simulink model "boggieDynamics2"  (R2022b)
settings: Solver=VariableStepAuto  StartTime=0.0  StopTime=10.0  RelTol=1e-3
values from neighbouring files (symbols this model uses):
  cg_nom = 0.567    [linealizacion_5gdl.m]    (also in linealizacion_HEMS.m)
undefined symbols (not defined in the file or in its folder): g, m, x_lev, x_lim, y_brk, y_lev, y_lim, z_brk, z_lev, z_lim
libraries: shared6dof x1
settings Model: Creator=USUARIO  LastModifiedBy=USUARIO

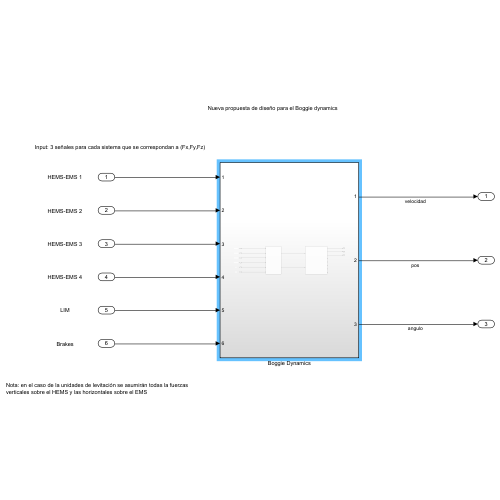
[thumbnail: Simulink's stored preview of the top-level diagram]
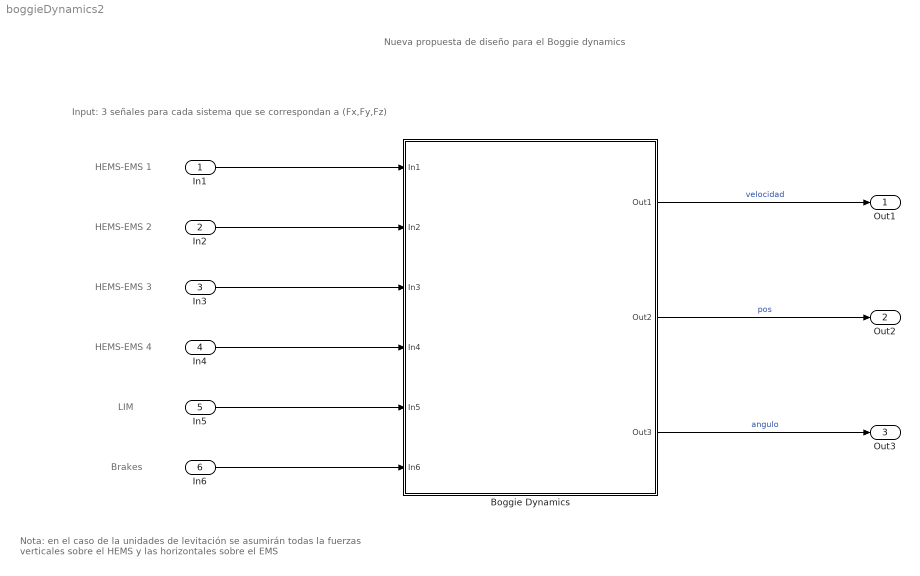
== system boggieDynamics2 ==
  note: Input: 3 señales para cada sistema que se correspondan a (Fx,Fy,Fz)
  note: Nueva propuesta de diseño para el Boggie dynamics
  note: HEMS-EMS 3
  note: Brakes
  note: HEMS-EMS 1
  note: LIM
  note: HEMS-EMS 4
  note: HEMS-EMS 2
  note: Nota: en el caso de la unidades de levitación se asumirán todas la fuerzas
      | verticales sobre el HEMS y las horizontales sobre el EMS
  In1 : Inport
  In2 : Inport  Port=2
  In3 : Inport  Port=3
  In4 : Inport  Port=4
  In5 : Inport  Port=5
  In6 : Inport  Port=6
  Boggie Dynamics : Subsystem
  Out1 : Outport
  Out2 : Outport  Port=2
  Out3 : Outport  Port=3
  wires:
  Boggie Dynamics/2(Out2) -> Out2/1  "pos"
  Boggie Dynamics/3(Out3) -> Out3/1  "angulo"
  Boggie Dynamics/1(Out1) -> Out1/1  "velocidad"
  In6/1 -> Boggie Dynamics/6(In6)
  In3/1 -> Boggie Dynamics/3(In3)
  In4/1 -> Boggie Dynamics/4(In4)
  In2/1 -> Boggie Dynamics/2(In2)
  In1/1 -> Boggie Dynamics/1(In1)
  In5/1 -> Boggie Dynamics/5(In5)

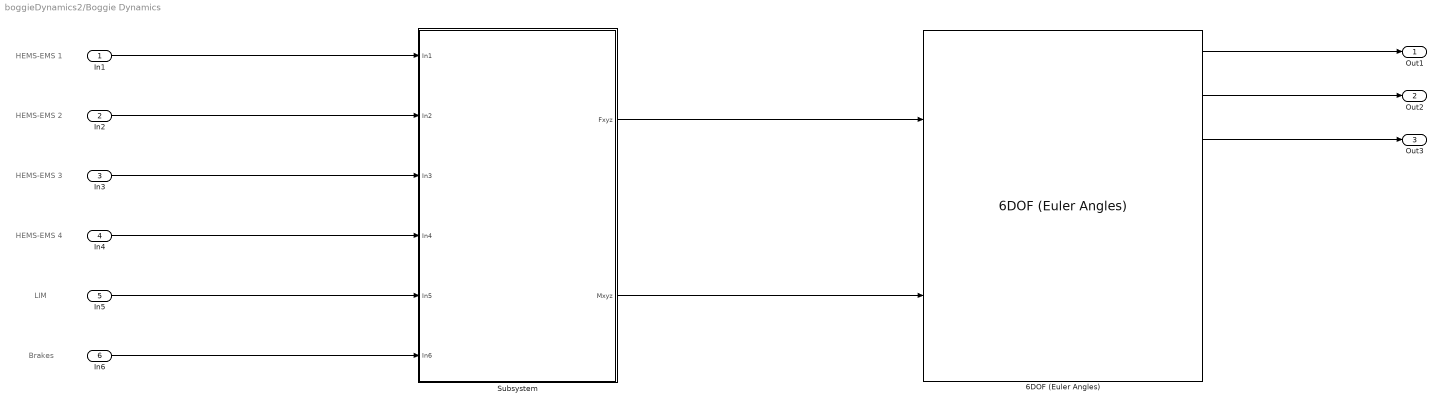
== system boggieDynamics2/Boggie Dynamics ==
  note: LIM
  note: HEMS-EMS 1
  note: HEMS-EMS 2
  note: HEMS-EMS 3
  note: HEMS-EMS 4
  note: Brakes
  In1 : Inport
  In2 : Inport  Port=2
  In3 : Inport  Port=3
  In4 : Inport  Port=4
  In5 : Inport  Port=5
  In6 : Inport  Port=6
  6DOF (Euler Angles) : shared6dof/6DOF (Euler Angles)  units=Metric (MKS)  mtype=Fixed  rep=Euler Angles  xme_0=[0 0 cg_nom]  Vm_0=[0 0 0]  eul_0=[0 0 0]  pm_0=[0 0 0]  mass_0=m  mass_e=0.5  mass_f=2.0  inertia=I  inertia_e=eye(3)  inertia_f=2*eye(3)  k_quat=1.0  vre_flag=on  abi_flag=off  aMode=0  xme_statename=''  Vm_statename=''  eul_statename=''  quat_statename=''  pm_statename=''  mass_statename=''
  Subsystem : Subsystem
  Out1 : Outport
  Out2 : Outport  Port=2
  Out3 : Outport  Port=3
  wires:
  6DOF (Euler Angles)/1 -> Out1/1
  6DOF (Euler Angles)/2 -> Out2/1
  6DOF (Euler Angles)/3 -> Out3/1
  In1/1 -> Subsystem/1(In1)
  In2/1 -> Subsystem/2(In2)
  In3/1 -> Subsystem/3(In3)
  In4/1 -> Subsystem/4(In4)
  In5/1 -> Subsystem/5(In5)
  In6/1 -> Subsystem/6(In6)
  Subsystem/1(Fxyz) -> 6DOF (Euler Angles)/1
  Subsystem/2(Mxyz) -> 6DOF (Euler Angles)/2

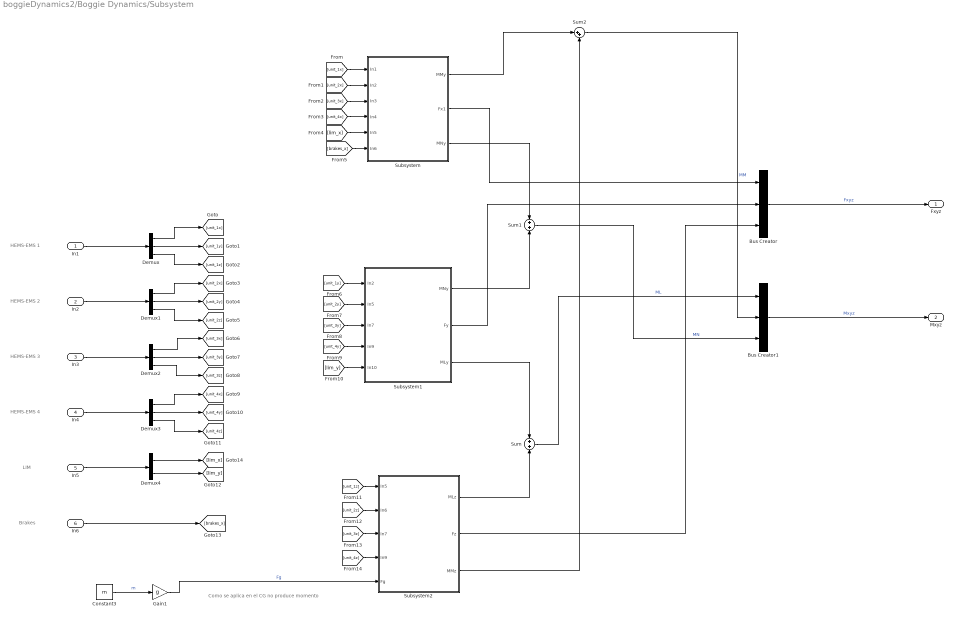
== system boggieDynamics2/Boggie Dynamics/Subsystem ==
  note: Como se aplica en el CG no produce momento
  note: HEMS-EMS 3
  note: Brakes
  note: HEMS-EMS 1
  note: LIM
  note: HEMS-EMS 4
  note: HEMS-EMS 2
  In1 : Inport
  In2 : Inport  Port=2
  In3 : Inport  Port=3
  In4 : Inport  Port=4
  In5 : Inport  Port=5
  In6 : Inport  Port=6
  Bus Creator : BusCreator  Inputs=3
  Bus Creator1 : BusCreator  Inputs=3
  Constant3 : Constant  Value=m
  Demux{,1..3} (4 alike) : Demux  Outputs=3
  Demux4 : Demux  Outputs=2
  Gain1 : Gain  Gain=g
  Subsystem : Subsystem
  Subsystem1 : Subsystem
  Subsystem2 : Subsystem
  Sum : Sum
  Sum1 : Sum
  Sum2 : Sum  Inputs=|++
  Fxyz : Outport
  Mxyz : Outport  Port=2
  wires:
  In3/1 -> Demux2/1
  Constant3/1 -> Gain1/1  "m"
  Sum2/1 -> Bus Creator1/2  "MM"
  Bus Creator/1 -> Fxyz/1  "Fxyz"
  In4/1 -> Demux3/1
  Bus Creator1/1 -> Mxyz/1  "Mxyz"
  Sum1/1 -> Bus Creator1/3  "MN"
  Sum/1 -> Bus Creator1/1  "ML"
  In2/1 -> Demux1/1
  In5/1 -> Demux4/1
  In6/1 -> [brakes_x]
  In1/1 -> Demux/1
  Subsystem/1(MMy) -> Sum2/1
  Subsystem/2(Fx1) -> Bus Creator/1
  Subsystem/3(MNy) -> Sum1/1
  Subsystem1/2(Fy) -> Bus Creator/2
  Subsystem1/1(MNy) -> Sum1/2
  Subsystem1/3(MLy) -> Sum/1
  Gain1/1 -> Subsystem2/5(Fg)  "Fg"
  Subsystem2/2(Fz) -> Bus Creator/3
  Subsystem2/1(MLz) -> Sum/2
  Demux4/2 -> [lim_y]
  Demux4/1 -> [lim_x]
  Demux3/1 -> [unit_4x]
  Demux3/2 -> [unit_4y]
  Demux3/3 -> [unit_4z]
  Demux2/1 -> [unit_3x]
  Demux2/2 -> [unit_3y]
  Demux2/3 -> [unit_3z]
  Demux1/1 -> [unit_2x]
  Demux1/2 -> [unit_2y]
  Demux1/3 -> [unit_2z]
  Demux/1 -> [unit_1x]
  Demux/2 -> [unit_1y]
  Demux/3 -> [unit_1z]
  Subsystem2/3(MMz) -> Sum2/2
  [unit_1x] -> Subsystem/1(In1)
  [unit_2x] -> Subsystem/2(In2)
  [unit_3x] -> Subsystem/3(In3)
  [unit_4x] -> Subsystem/4(In4)
  [lim_x] -> Subsystem/5(In5)
  [brakes_x] -> Subsystem/6(In6)
  [unit_4y] -> Subsystem1/4(In9)
  [unit_1y] -> Subsystem1/1(In2)
  [lim_y] -> Subsystem1/5(In10)
  [unit_2y] -> Subsystem1/2(In5)
  [unit_3y] -> Subsystem1/3(In7)
  [unit_1z] -> Subsystem2/1(In5)
  [unit_3z] -> Subsystem2/3(In7)
  [unit_2z] -> Subsystem2/2(In6)
  [unit_4z] -> Subsystem2/4(In9)

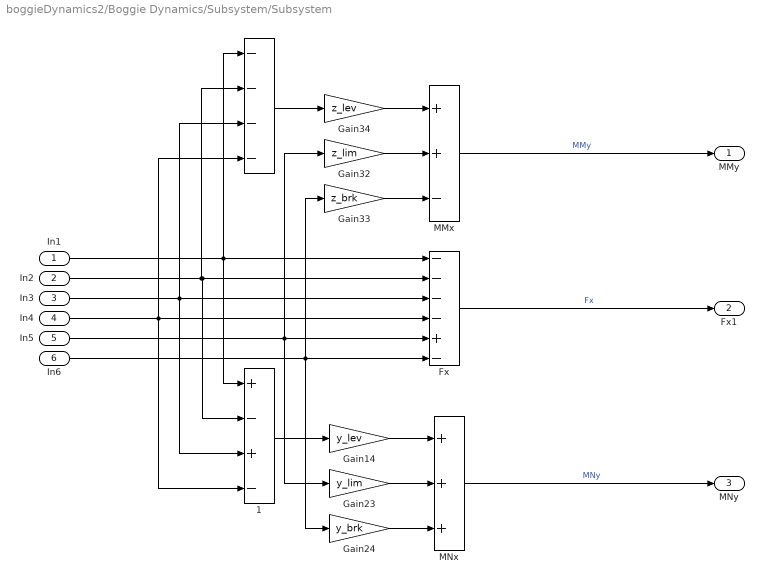
== system boggieDynamics2/Boggie Dynamics/Subsystem/Subsystem ==
  In1 : Inport
  In2 : Inport  Port=2
  In3 : Inport  Port=3
  In4 : Inport  Port=4
  In5 : Inport  Port=5
  In6 : Inport  Port=6
  " " : Sum  Inputs=----
  " 1" : Sum  Inputs=+-+-
  Fx : Sum  Inputs=----+-
  Gain14 : Gain  Gain=y_lev
  Gain23 : Gain  Gain=y_lim
  Gain24 : Gain  Gain=y_brk
  Gain32 : Gain  Gain=z_lim
  Gain33 : Gain  Gain=z_brk
  Gain34 : Gain  Gain=z_lev
  MMx : Sum  Inputs=++-
  MNx : Sum  Inputs=+++
  MMy : Outport
  Fx1 : Outport  Port=2
  MNy : Outport  Port=3
  wires:
  In1/1 -> " 1"/1, " "/1, Fx/1
  In2/1 -> " "/2, " 1"/2, Fx/2
  Fx/1 -> Fx1/1  "Fx"
  MMx/1 -> MMy/1  "MMy"
  In4/1 -> " "/4, Fx/4, " 1"/4
  In6/1 -> Gain24/1, Fx/6, Gain33/1
  In5/1 -> Gain23/1, Gain32/1, Fx/5
  In3/1 -> " 1"/3, " "/3, Fx/3
  Gain32/1 -> MMx/2
  Gain34/1 -> MMx/1
  Gain33/1 -> MMx/3
  Gain14/1 -> MNx/1
  MNx/1 -> MNy/1  "MNy"
  " "/1 -> Gain34/1
  Gain24/1 -> MNx/3
  Gain23/1 -> MNx/2
  " 1"/1 -> Gain14/1

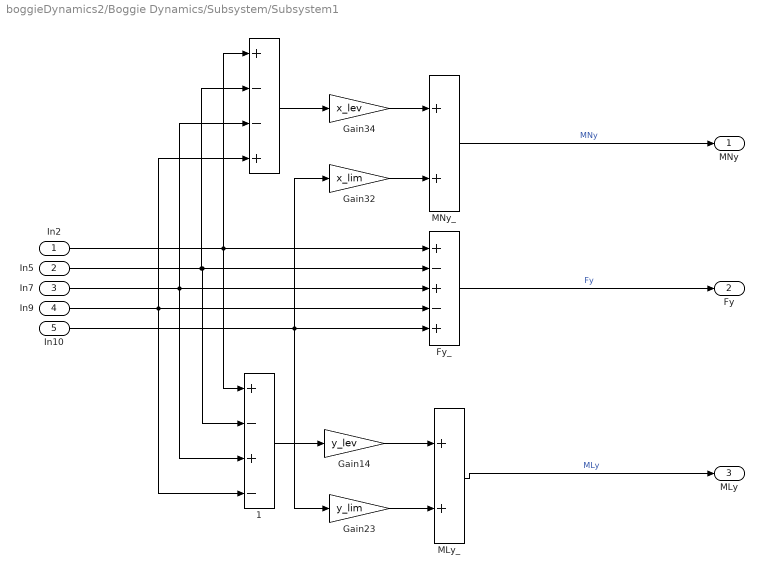
== system boggieDynamics2/Boggie Dynamics/Subsystem/Subsystem1 ==
  In2 : Inport
  In5 : Inport  Port=2
  In7 : Inport  Port=3
  In9 : Inport  Port=4
  In10 : Inport  Port=5
  " " : Sum  Inputs=+--+
  " 1" : Sum  Inputs=+-+-
  Fy_ : Sum  Inputs=+-+-+
  Gain14 : Gain  Gain=y_lev
  Gain23 : Gain  Gain=y_lim
  Gain32 : Gain  Gain=x_lim
  Gain34 : Gain  Gain=x_lev
  MLy_ : Sum
  MNy_ : Sum
  MNy : Outport
  Fy : Outport  Port=2
  MLy : Outport  Port=3
  wires:
  " 1"/1 -> Gain14/1
  " "/1 -> Gain34/1
  Fy_/1 -> Fy/1  "Fy"
  MLy_/1 -> MLy/1  "MLy"
  Gain32/1 -> MNy_/2
  Gain14/1 -> MLy_/1
  Gain34/1 -> MNy_/1
  In7/1 -> " 1"/3, Fy_/3, " "/3
  In9/1 -> " 1"/4, Fy_/4, " "/4
  In2/1 -> " 1"/1, Fy_/1, " "/1
  In5/1 -> " "/2, " 1"/2, Fy_/2
  MNy_/1 -> MNy/1  "MNy"
  In10/1 -> Gain32/1, Gain23/1, Fy_/5
  Gain23/1 -> MLy_/2

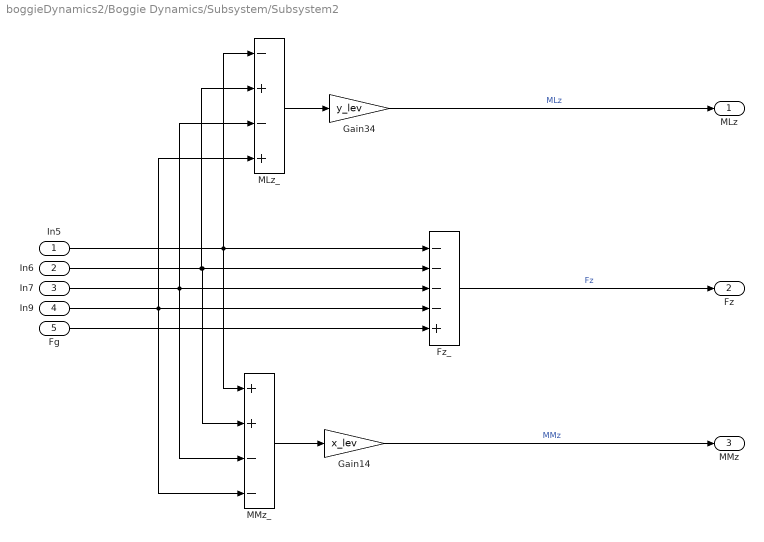
== system boggieDynamics2/Boggie Dynamics/Subsystem/Subsystem2 ==
  In5 : Inport
  In6 : Inport  Port=2
  In7 : Inport  Port=3
  In9 : Inport  Port=4
  Fg : Inport  Port=5
  " MLz_" : Sum  Inputs=-+-+
  Fz_ : Sum  Inputs=----+
  Gain14 : Gain  Gain=x_lev
  Gain34 : Gain  Gain=y_lev
  MMz_ : Sum  Inputs=++--
  MLz : Outport
  Fz : Outport  Port=2
  MMz : Outport  Port=3
  wires:
  In6/1 -> " MLz_"/2, MMz_/2, Fz_/2
  Gain34/1 -> MLz/1  "MLz"
  Fg/1 -> Fz_/5
  In9/1 -> MMz_/4, Fz_/4, " MLz_"/4
  In5/1 -> MMz_/1, Fz_/1, " MLz_"/1
  In7/1 -> MMz_/3, Fz_/3, " MLz_"/3
  MMz_/1 -> Gain14/1
  " MLz_"/1 -> Gain34/1
  Fz_/1 -> Fz/1  "Fz"
  Gain14/1 -> MMz/1  "MMz"
